simulink model "derivative"  (R2022a)
settings: Solver=VariableStepAuto  StartTime=0.0  StopTime=10.0  RelTol=1e-3
values from neighbouring files (symbols this model uses):
  samplederivative = 0.025    [parametros.m]
libraries: simulink x2
settings Model: Creator=Franciele Sembay  LastModifiedBy=Franciele Sembay

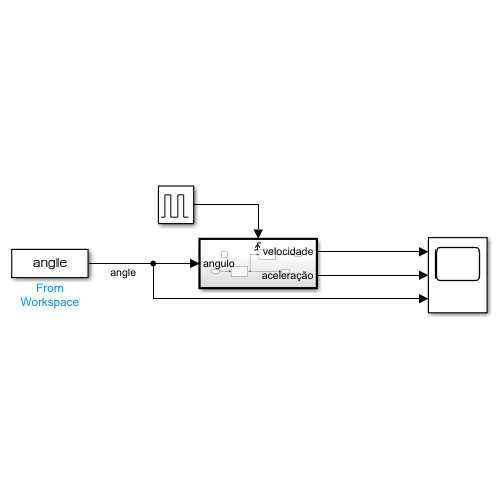
[thumbnail: Simulink's stored preview of the top-level diagram]
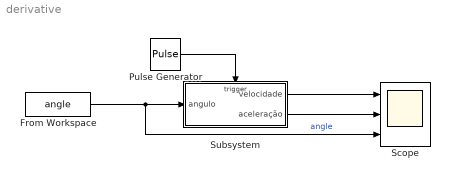
== system derivative ==
  From Workspace : FromWorkspace  VariableName=angle  OutputAfterFinalValue=Holding final value
  Pulse Generator : DiscretePulseGenerator  PulseType=Time based  Period=samplederivative  PulseWidth=50  PhaseDelay=samplederivative
  Scope : Scope  NumInputPorts=3
  Subsystem : Subsystem
  wires:
  Subsystem/2(aceleração) -> Scope/2
  From Workspace/1 -> Scope/3, Subsystem/1(angulo)  "angle"
  Pulse Generator/1 -> Subsystem/Trigger
  Subsystem/1(velocidade) -> Scope/1

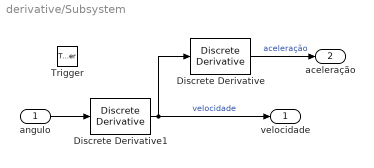
== system derivative/Subsystem ==
  angulo : Inport
  Trigger : TriggerPort  VariantControl=(inherit)  InitialTriggerSignalState=zero  PortDimensions=1
  Discrete Derivative : simulink/Discrete/Discrete Derivative  gainval=1.0  ICPrevScaledInput=0.0  OutMin=[]  OutMax=[]  OutDataType=fixdt(1, 16)  OutScaling=2^-10  DoSatur=off
  Discrete Derivative1 : simulink/Discrete/Discrete Derivative  gainval=1.0  ICPrevScaledInput=0.0  OutMin=[]  OutMax=[]  OutDataType=fixdt(1, 16)  OutScaling=2^-10  DoSatur=off
  velocidade : Outport
  aceleração : Outport  Port=2
  wires:
  angulo/1 -> Discrete Derivative1/1
  Discrete Derivative1/1 -> Discrete Derivative/1, velocidade/1  "velocidade"
  Discrete Derivative/1 -> aceleração/1  "aceleração"
